simulink model "inverter_16"  (R2016a)
settings: Solver=VariableStepAuto  SolverMode=SingleTasking  StartTime=0.0  StopTime=0.1  MaxStep=1e-4  RelTol=1e-3
libraries: powerlib x33, powerlib_meascontrol x3
settings Model: Creator=narendra  LastModifiedBy=narendra
settings DebuggingCC: SFUnexpectedBacktrackingDiag=error  SFNoUnconditionalDefaultTransitionDiag=error
settings GRTTargetCC: TargetLangStandard=C99 (ISO)  GeneratePreprocessorConditionals=Use local settings
settings ConfigComp: CovMetricSettings=dwe  CovHtmlReporting=off  CovSaveCumulativeToWorkspaceVar=off  CovSaveSingleToWorkspaceVar=off  CovExternalEMLEnable=on

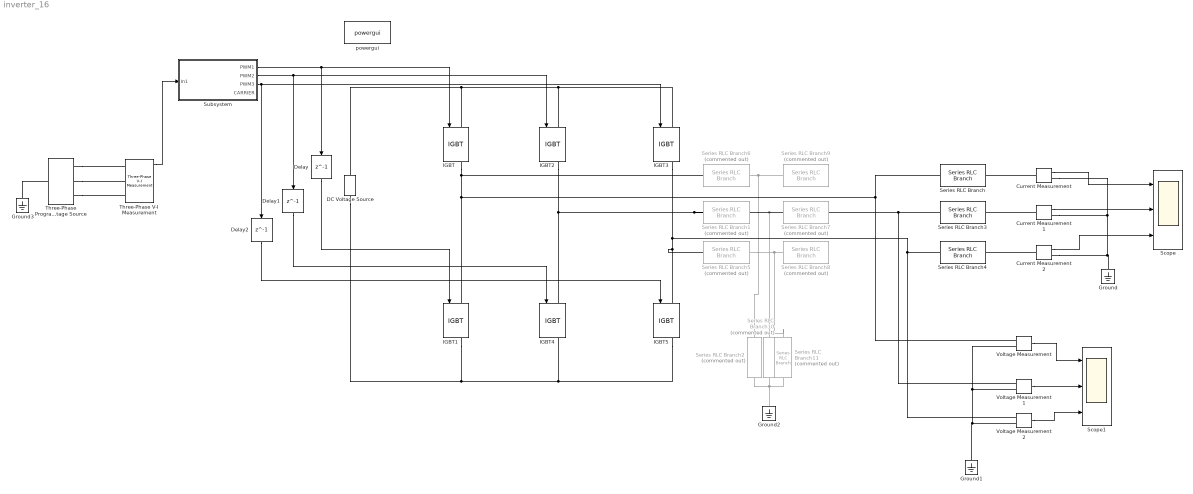
== system inverter_16 ==
  Current Measurement : powerlib/Measurements/Current Measurement  PhasorSimulation=off  OutputType=Complex  PSBequivalent=0
  Current Measurement1 : powerlib/Measurements/Current Measurement  PhasorSimulation=off  OutputType=Complex  PSBequivalent=0
  Current Measurement2 : powerlib/Measurements/Current Measurement  PhasorSimulation=off  OutputType=Complex  PSBequivalent=0
  DC Voltage Source : powerlib/Electrical Sources/DC Voltage Source  Amplitude=200  Measurements=None
  Delay : Delay  DelayLength=1  InitialCondition=0
  Delay1 : Delay  DelayLength=1  InitialCondition=0
  Delay2 : Delay  DelayLength=1  InitialCondition=0
  Ground{,1..3} (4 alike) : powerlib/Elements/Ground  LConnTagsString=a
  IGBT{,1..5} (6 alike) : powerlib/Power Electronics/IGBT  Ron=0.001  Lon=0  Vf=1  Tf=1e-6  Tt=2e-6  IC=0  Rs=1e5  Cs=inf  Measurements=on
  Scope : Scope  NumInputPorts=3
  Scope1 : Scope  NumInputPorts=3
  Series RLC Branch : powerlib/Elements/Series RLC Branch  LConnTagsString=__new0  RConnTagsString=__new0  BranchType=R  Resistance=10  Inductance=1e-3  SetiL0=off  InitialCurrent=0  Capacitance=1e-6  Setx0=off  InitialVoltage=0  Measurements=None
  Series RLC Branch1 : powerlib/Elements/Series RLC Branch  Commented=on  LConnTagsString=__new0  RConnTagsString=__new0  BranchType=L  Resistance=1  Inductance=0.08  SetiL0=off  InitialCurrent=0  Capacitance=1e-6  Setx0=off  InitialVoltage=0  Measurements=None
  Series RLC Branch10 : powerlib/Elements/Series RLC Branch  Commented=on  LConnTagsString=__new0  RConnTagsString=__new0  BranchType=C  Resistance=1  Inductance=1e-3  SetiL0=off  InitialCurrent=0  Capacitance=50e-6  Setx0=off  InitialVoltage=0  Measurements=None
  Series RLC Branch11 : powerlib/Elements/Series RLC Branch  Commented=on  LConnTagsString=__new0  RConnTagsString=__new0  BranchType=C  Resistance=1  Inductance=1e-3  SetiL0=off  InitialCurrent=0  Capacitance=50e-6  Setx0=off  InitialVoltage=0  Measurements=None
  Series RLC Branch2 : powerlib/Elements/Series RLC Branch  Commented=on  LConnTagsString=__new0  RConnTagsString=__new0  BranchType=C  Resistance=1  Inductance=1e-3  SetiL0=off  InitialCurrent=0  Capacitance=50e-6  Setx0=off  InitialVoltage=0  Measurements=None
  Series RLC Branch3 : powerlib/Elements/Series RLC Branch  LConnTagsString=__new0  RConnTagsString=__new0  BranchType=R  Resistance=10  Inductance=1e-3  SetiL0=off  InitialCurrent=0  Capacitance=1e-6  Setx0=off  InitialVoltage=0  Measurements=None
  Series RLC Branch4 : powerlib/Elements/Series RLC Branch  LConnTagsString=__new0  RConnTagsString=__new0  BranchType=R  Resistance=10  Inductance=1e-3  SetiL0=off  InitialCurrent=0  Capacitance=1e-6  Setx0=off  InitialVoltage=0  Measurements=None
  Series RLC Branch5 : powerlib/Elements/Series RLC Branch  Commented=on  LConnTagsString=__new0  RConnTagsString=__new0  BranchType=L  Resistance=1  Inductance=0.08  SetiL0=off  InitialCurrent=0  Capacitance=1e-6  Setx0=off  InitialVoltage=0  Measurements=None
  Series RLC Branch6 : powerlib/Elements/Series RLC Branch  Commented=on  LConnTagsString=__new0  RConnTagsString=__new0  BranchType=L  Resistance=1  Inductance=0.08  SetiL0=off  InitialCurrent=0  Capacitance=1e-6  Setx0=off  InitialVoltage=0  Measurements=None
  Series RLC Branch7 : powerlib/Elements/Series RLC Branch  Commented=on  LConnTagsString=__new0  RConnTagsString=__new0  BranchType=L  Resistance=1  Inductance=0.06  SetiL0=off  InitialCurrent=0  Capacitance=1e-6  Setx0=off  InitialVoltage=0  Measurements=None
  Series RLC Branch8 : powerlib/Elements/Series RLC Branch  Commented=on  LConnTagsString=__new0  RConnTagsString=__new0  BranchType=L  Resistance=1  Inductance=0.06  SetiL0=off  InitialCurrent=0  Capacitance=1e-6  Setx0=off  InitialVoltage=0  Measurements=None
  Series RLC Branch9 : powerlib/Elements/Series RLC Branch  Commented=on  LConnTagsString=__new0  RConnTagsString=__new0  BranchType=L  Resistance=1  Inductance=0.06  SetiL0=off  InitialCurrent=0  Capacitance=1e-6  Setx0=off  InitialVoltage=0  Measurements=None
  Subsystem : Subsystem
  Three-Phase Programmable Voltage Source : powerlib/Electrical Sources/Three-Phase Programmable Voltage Source  PositiveSequence="[1  0 60]"  VariationEntity=None  VariationType=Table of time-amplitude pairs  VariationTypeAlt=Step  VariationStep=0.5  VariationRate=10  VariationMagnitude=0.3  VariationFrequency=2  VariationTiming=[1 2]  VariationPhaseA=off  Amplitudes=[1 0.8 1.2 1.0]  TimeValues=[0 0.1 0.15 0.2]  HarmonicGeneration=off  HarmonicA=[3 0.2 -25 0]  HarmonicB=[2 0.15 35 2]  Timing="[0.05  3]"  BusType=swing  Pref=0  Qref=0  Qmin=-inf  Qmax=inf
  Three-Phase V-I Measurement : powerlib/Measurements/Three-Phase V-I Measurement  VoltageMeasurement=phase-to-ground  SetLabelV=off  LabelV=Vabc  Vpu=off  VpuLL=off  CurrentMeasurement=yes  SetLabelI=off  LabelI=Iabc  Ipu=off  Pbase=100e6  Vbase=500e3  OutputType=Complex  PhasorSimulation=off  PSBequivalent=0
  Voltage Measurement : powerlib/Measurements/Voltage Measurement  PhasorSimulation=off  OutputType=Complex  PSBequivalent=0
  Voltage Measurement1 : powerlib/Measurements/Voltage Measurement  PhasorSimulation=off  OutputType=Complex  PSBequivalent=0
  Voltage Measurement2 : powerlib/Measurements/Voltage Measurement  PhasorSimulation=off  OutputType=Complex  PSBequivalent=0
  powergui : powerlib/powergui  Priority=1  SimulationMode=Continuous  SampleTime=50e-6  frequency=60  Iterations=50  frequencyindice=0  Pbase=100e6  ErrMax=1e-4  UnitsV=kV  UnitsW=MW  buscounter=0  FunctionMessages=off  echomessages=off  EnableUseOfTLC=off  CurrentSourceSwitches=off  DisableSnubberDevices=off  DisableRonSwitches=off  DisableVfSwitches=off  DisplayEquations=off  SolverType=Tustin/Backward Euler (TBE)  Interpol=off  ExternalGateDelay=off  methode=off  Ts=100  x0status=blocks  SPID=on  SwTol=0  HookPort=off  RestoreLinks=warning  ResistiveCurrentMeasurement=off  Frange=[0:2:500]  Ylog=off  Xlog=on  ShowGrid=off  save=off  variable=ZData  structure=0  ZoomFFT=off  StartTime=0.0  cycles=1  DisplayStyle=1  fundamental=60  FreqAxis=off  MaxFrequency=1000  frequencyindicesteady=1  RmsSteady=1  display=off
  wires:
  Subsystem/1(PWM1) -> Delay/1, IGBT/1
  Subsystem/2(PWM2) -> Delay1/1, IGBT2/1
  Subsystem/3(PWM3) -> Delay2/1, IGBT3/1
  Delay/1 -> IGBT1/1
  Delay1/1 -> IGBT4/1
  Delay2/1 -> IGBT5/1
  Voltage Measurement/1 -> Scope1/1
  Voltage Measurement1/1 -> Scope1/2
  Voltage Measurement2/1 -> Scope1/3
  Current Measurement/1 -> Scope/1
  Current Measurement1/1 -> Scope/2
  Current Measurement2/1 -> Scope/3
  Three-Phase V-I Measurement/1 -> Subsystem/1(In1)
  connections:
  IGBT/LConn1 -- DC Voltage Source/RConn1 -- IGBT3/LConn1 -- IGBT2/LConn1
  IGBT1/RConn1 -- DC Voltage Source/LConn1 -- IGBT5/RConn1 -- IGBT4/RConn1
  Current Measurement2/LConn1 -- Series RLC Branch4/RConn1
  Current Measurement1/LConn1 -- Series RLC Branch3/RConn1
  Current Measurement/LConn1 -- Series RLC Branch/RConn1
  Current Measurement2/RConn1 -- Current Measurement/RConn1 -- Current Measurement1/RConn1 -- Ground/LConn1
  Voltage Measurement/LConn2 -- Voltage Measurement1/LConn2 -- Voltage Measurement2/LConn2 -- Ground1/LConn1
  Series RLC Branch9/LConn1 -- Series RLC Branch2/LConn1 -- Series RLC Branch6/RConn1
  Series RLC Branch1/RConn1 -- Series RLC Branch10/LConn1 -- Series RLC Branch7/LConn1
  Series RLC Branch5/RConn1 -- Series RLC Branch11/LConn1 -- Series RLC Branch8/LConn1
  Series RLC Branch2/RConn1 -- Ground2/LConn1 -- Series RLC Branch11/RConn1 -- Series RLC Branch10/RConn1
  IGBT2/RConn1 -- Series RLC Branch1/LConn1 -- Voltage Measurement1/LConn1 -- Series RLC Branch3/LConn1 -- IGBT4/LConn1
  IGBT/RConn1 -- Series RLC Branch6/LConn1 -- Series RLC Branch/LConn1 -- Voltage Measurement/LConn1 -- IGBT1/LConn1
  IGBT3/RConn1 -- Series RLC Branch5/LConn1 -- IGBT5/LConn1 -- Series RLC Branch4/LConn1 -- Voltage Measurement2/LConn1
  Three-Phase Programmable Voltage Source/RConn1 -- Three-Phase V-I Measurement/LConn1
  Three-Phase Programmable Voltage Source/RConn2 -- Three-Phase V-I Measurement/LConn2
  Three-Phase Programmable Voltage Source/RConn3 -- Three-Phase V-I Measurement/LConn3
  Ground3/LConn1 -- Three-Phase Programmable Voltage Source/LConn1

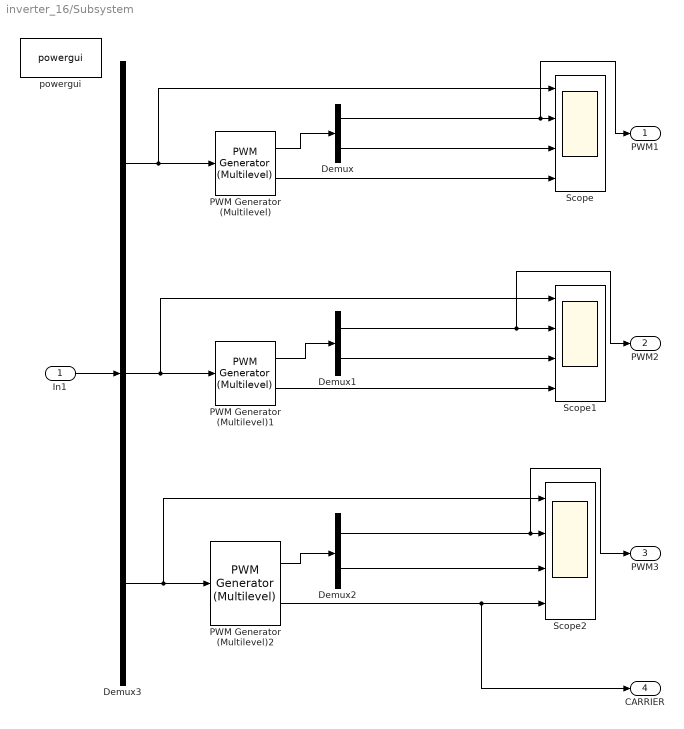
== system inverter_16/Subsystem ==
  In1 : Inport
  Demux : Demux  Outputs=2
  Demux1 : Demux  Outputs=2
  Demux2 : Demux  Outputs=2
  Demux3 : Demux  Outputs=3
  PWM Generator (Multilevel) : powerlib_meascontrol/Pulse & Signal Generators/PWM Generator (Multilevel)  BridgeType=Half-bridge  NumberOfBridges=1  Fc=20000  Ts=0  ShowCarriersOutport=on
  PWM Generator (Multilevel)1 : powerlib_meascontrol/Pulse & Signal Generators/PWM Generator (Multilevel)  BridgeType=Half-bridge  NumberOfBridges=1  Fc=20000  Ts=0  ShowCarriersOutport=on
  PWM Generator (Multilevel)2 : powerlib_meascontrol/Pulse & Signal Generators/PWM Generator (Multilevel)  BridgeType=Half-bridge  NumberOfBridges=1  Fc=20000  Ts=0  ShowCarriersOutport=on
  Scope : Scope  NumInputPorts=4
  Scope1 : Scope  NumInputPorts=4
  Scope2 : Scope  NumInputPorts=4
  powergui : powerlib/powergui  Priority=1  SimulationMode=Continuous  SampleTime=50e-6  frequency=60  Iterations=50  frequencyindice=60  Pbase=100e6  ErrMax=1e-4  UnitsV=kV  UnitsW=MW  buscounter=0  FunctionMessages=off  echomessages=off  EnableUseOfTLC=off  CurrentSourceSwitches=off  DisableSnubberDevices=off  DisableRonSwitches=off  DisableVfSwitches=off  DisplayEquations=off  SolverType=Tustin/Backward Euler (TBE)  Interpol=off  ExternalGateDelay=off  methode=off  Ts=100  x0status=blocks  SPID=on  SwTol=0  HookPort=off  RestoreLinks=warning  ResistiveCurrentMeasurement=off  Frange=[0:2:500]  Ylog=off  Xlog=on  ShowGrid=off  save=off  variable=ZData  structure=0  ZoomFFT=off  StartTime=0.0  cycles=1  DisplayStyle=1  fundamental=60  FreqAxis=off  MaxFrequency=1000  frequencyindicesteady=1  RmsSteady=1  display=off
  PWM1 : Outport
  PWM2 : Outport  Port=2
  PWM3 : Outport  Port=3
  CARRIER : Outport  Port=4
  wires:
  In1/1 -> Demux3/1
  Demux3/1 -> Scope/1, PWM Generator (Multilevel)/1
  Demux3/3 -> PWM Generator (Multilevel)2/1, Scope2/1
  Demux2/1 -> PWM3/1, Scope2/2
  PWM Generator (Multilevel)1/1 -> Demux1/1
  Demux1/1 -> PWM2/1, Scope1/2
  PWM Generator (Multilevel)1/2 -> Scope1/4
  Demux1/2 -> Scope1/3
  PWM Generator (Multilevel)/2 -> Scope/4
  Demux/2 -> Scope/3
  PWM Generator (Multilevel)/1 -> Demux/1
  Demux/1 -> PWM1/1, Scope/2
  Demux3/2 -> PWM Generator (Multilevel)1/1, Scope1/1
  Demux2/2 -> Scope2/3
  PWM Generator (Multilevel)2/2 -> Scope2/4, CARRIER/1
  PWM Generator (Multilevel)2/1 -> Demux2/1
